simulink model "rpoco8_100_r2"  (R2013a)
settings: Solver=VariableStepDiscrete  SolverMode=SingleTasking  StartTime=0.0  StopTime=10.0  RelTol=1e-3
libraries: xbsIndex_r4 x2263, casper_library_misc x52, casper_library_multipliers x19, xps_library x5, casper_library_sources x4, casper_library_delays x1
(part 3 of 27)

== system rpoco8_100_r2/eq_fft3 ==
  note: Slice out 6 MSb of addr counter
      | to select 32 coeffs per antenna's (2) N fft bins
  pol1 : Inport
  sync : Inport  Port=2
  coeff : Inport  Port=3
  coeff_we : Inport  Port=4
  coeff_addr : Inport  Port=5
  Constant4 : xbsIndex_r4/Constant  const=0  gui_display_data_type=Fixed-point  arith_type=Unsigned  n_bits=17  bin_pt=7  preci_type=Single  exp_width=8  frac_width=24  explicit_period=on  period=1  equ=P=C  opselect=C  inp2=PCIN>>17  opr=+  inp1=P  carry=CIN  dbl_ovrd=off  block_type=constant
  Constant5 : xbsIndex_r4/Constant  const=0  gui_display_data_type=Fixed-point  arith_type=Boolean  n_bits=1  bin_pt=0  preci_type=Single  exp_width=8  frac_width=24  explicit_period=on  period=1  equ=P=C  opselect=C  inp2=PCIN>>17  opr=+  inp1=P  carry=CIN  dbl_ovrd=off  block_type=constant
  Counter2 : xbsIndex_r4/Counter  cnt_type=Free Running  cnt_to=Inf  operation=Up  start_count=0  cnt_by_val=1  arith_type=Unsigned  n_bits=nchan  bin_pt=0  load_pin=off  rst=on  en=off  explicit_period=off  period=1  dbl_ovrd=off  use_behavioral_HDL=off  implementation=Fabric  use_rpm=on  block_type=counter
      settings: xl_area=[0, 0, 0, 0, 0, 0, 0]
  Delay11 : xbsIndex_r4/Delay  rst=off  infoeditControl=Selection of Reset will increase slice count due to use of real FFs and instead of SRLs  en=off  latency=2  dbl_ovrd=off  reg_retiming=off  block_type=delay
      settings: xl_area=[0, 0, 0, 0, 0, 0, 0]
  Delay4 : xbsIndex_r4/Delay  rst=off  infoeditControl=Selection of Reset will increase slice count due to use of real FFs and instead of SRLs  en=off  latency=7  dbl_ovrd=off  reg_retiming=off  block_type=delay
      settings: xl_area=[0, 0, 0, 0, 0, 0, 0]
  Dual Port RAM : xbsIndex_r4/Dual Port RAM  depth=2^6  initVector=0  distributed_mem=Block RAM  init_a=0  init_b=0  rst_a=off  rst_b=off  en_a=off  en_b=off  latency=2  write_mode_A=Read After Write  write_mode_B=Read After Write  dbl_ovrd=off  optimize=Area  block_type=dpram
      settings: xl_area=[0, 0, 0, 0, 0, 0, 0]  block_version=10.1.3
  Reinterpret1 : xbsIndex_r4/Reinterpret  force_arith_type=on  arith_type=Unsigned  force_bin_pt=on  bin_pt=7  block_type=reinterpret
      settings: infoedit="Changes signal type without altering the binary representation.   You can changed the signal between signed and unsigned, and relocate the binary point.<br><br>Hardware notes: In hardware this block costs nothing.<br><br>Example:  Suppose the input is 6 bits wide, signed, with 2 fractional bits, and the output is forced to unsigned with 0 fractional bits.  Then an input of -2.0 (1110.00 in binary 2's complement) becomes an output of 56 (111000 in binary)."  block_version=10.1.3
  Slice : xbsIndex_r4/Slice  nbits=6  boolean_output=off  mode=Upper Bit Location + Width  bit1=0  base1=MSB of Input  bit0=0  base0=LSB of Input  dbl_ovrd=off  block_type=slice
      settings: infoedit="Extracts a given range of bits from each input sample and presents it at the output.  The output type is ordinarily unsigned with binary point at zero, but can be Boolean when the slice is one bit wide.<P><P>Hardware notes: In hardware this block costs nothing."  block_version=10.1.3
  Terminator : Terminator
  round1 : Subsystem  mask{n_bits=18}
      mask prompts: n_bits "Output Bitwidth"
  dout : Outport
  sync_out : Outport  Port=2
  clip : Outport  Port=3
  wires:
  Constant4/1 -> Dual Port RAM/2
  Constant5/1 -> Dual Port RAM/3
  coeff_addr/1 -> Dual Port RAM/4
  coeff_we/1 -> Dual Port RAM/6
  Reinterpret1/1 -> Dual Port RAM/5
  sync/1 -> Counter2/1, Delay4/1
  coeff/1 -> Reinterpret1/1
  round1/1(dout) -> dout/1
  Delay11/1 -> round1/1(din)
  pol1/1 -> Delay11/1
  Delay4/1 -> sync_out/1
  round1/2(clip) -> clip/1
  Counter2/1 -> Slice/1
  Slice/1 -> Dual Port RAM/1
  Dual Port RAM/2 -> Terminator/1
  Dual Port RAM/1 -> round1/2(scale)

== system rpoco8_100_r2/fft_pol02_imag ==
  addr : Inport
  data_in : Inport  Port=2
  we : Inport  Port=3
  calc_add : Subsystem  mask{data_width=32, addr_width=11, sample_rate=sample_rate}
      mask prompts: data_width "data width"; addr_width "address width"; sample_rate "sample rate"
  convert_addr : xbsIndex_r4/Convert  gui_display_data_type=Fixed-point  arith_type=Unsigned  n_bits=addr_width  bin_pt=0  float_type=Single  exp_bits=8  fraction_bits=24  quantization=Truncate  overflow=Wrap  en=off  latency=0  dbl_ovrd=off  pipeline=off  block_type=convert
      settings: xl_area=[0, 0, 0, 0, 0, 0, 0]
  convert_din1 : xbsIndex_r4/Convert  gui_display_data_type=Fixed-point  arith_type=Unsigned  n_bits=32  bin_pt=0  float_type=Single  exp_bits=8  fraction_bits=24  quantization=Truncate  overflow=Wrap  en=off  latency=0  dbl_ovrd=off  pipeline=off  block_type=convert
      settings: xl_area=[0, 0, 0, 0, 0, 0, 0]
  convert_we : xbsIndex_r4/Convert  gui_display_data_type=Fixed-point  arith_type=Unsigned  n_bits=1  bin_pt=0  float_type=Single  exp_bits=8  fraction_bits=24  quantization=Truncate  overflow=Wrap  en=off  latency=0  dbl_ovrd=off  pipeline=off  block_type=convert
      settings: xl_area=[0, 0, 0, 0, 0, 0, 0]
  mem : Subsystem
  munge_in : Subsystem  AncestorBlock=casper_library_flow_control/munge  mask(munge){divisions=1, div_size=32, order=[0], arith_type_out=Unsigned, bin_pt_out=0}
      mask prompts: divisions "Number of divisions"; div_size "Division size (bits)"; order "Division packing order"; arith_type_out "Output arithmetic type"; bin_pt_out "Output binary point"
      mask help: Splits an input bus into the specified number of divisions and then recombines them in the order specified (most significant division = 0,least = number divisions-1)
      mask init:
      | munge_init(gcb, ...
      |     'divisions', divisions, ...
      |     'div_size', div_size, ...
      |     'order', order, ...
      |     'arith_type_out', arith_type_out, ...
      |     'bin_pt_out', bin_pt_out);
      settings: AttributesFormatString=|
      | split:32
      | join:0
      | Unsigned [32,0]
      mask TypeOptions arith_type_out: Unsigned | Signed  (2's comp) | Floating-point
  munge_out : Subsystem  AncestorBlock=casper_library_flow_control/munge  mask(munge){divisions=1, div_size=32, order=[0], arith_type_out=Unsigned, bin_pt_out=0}
      mask prompts: divisions "Number of divisions"; div_size "Division size (bits)"; order "Division packing order"; arith_type_out "Output arithmetic type"; bin_pt_out "Output binary point"
      mask help: Splits an input bus into the specified number of divisions and then recombines them in the order specified (most significant division = 0,least = number divisions-1)
      mask init:
      | munge_init(gcb, ...
      |     'divisions', divisions, ...
      |     'div_size', div_size, ...
      |     'order', order, ...
      |     'arith_type_out', arith_type_out, ...
      |     'bin_pt_out', bin_pt_out);
      settings: AttributesFormatString=|
      | split:32
      | join:0
      | Unsigned [32,0]
      mask TypeOptions arith_type_out: Unsigned | Signed  (2's comp) | Floating-point
  rpoco8_r2_fft_pol02_imag_addr : xbsIndex_r4/Gateway Out  inherit_from_input=off  hdl_port=on  timing_constraint=None  locs_specified=off  LOCs={'A5','B9','A9','C1','A3','G6','E9','A6','A7','A8','B8','B1','B3','D9','B5','B4','B6','C2'}  UseAsDAC=off  DACChannel='1'  block_type=gatewayout
      settings: infoedit="Gateway out block.  Converts Xilinx fixed point inputs into ouputs of type Simulink integer, double, or fixed point.<P><P>Hardware notes:  In hardware these blocks become top level output ports or are discarded, depending on how they are configured."  xl_area=[0, 0, 0, 0, 0, 0, 0]  sginterface={'Nallatech'=>{'xdspkit'=>{'non_memory_mapped_port'=>'uprev_Shared_BRAM_addr'}},'Xilinx'=>{'jtaghwcosim'=>{'non_memory_mapped_port'=>'uprev_Shared_BRAM_addr'},'xdspkit'=>{'non_memory_mapped_port'=>'uprev_Shared_BRAM_addr'}}}
  rpoco8_r2_fft_pol02_imag_data_in : xbsIndex_r4/Gateway Out  inherit_from_input=off  hdl_port=on  timing_constraint=None  locs_specified=off  LOCs={'B21','B22','A22','B23','B19','C19','A20','A21','A23','B24','A24','A25','E18','D18','C18','B18'}  UseAsDAC=off  DACChannel='1'  block_type=gatewayout
      settings: infoedit="Gateway out block.  Converts Xilinx fixed point inputs into ouputs of type Simulink integer, double, or fixed point.<P><P>Hardware notes:  In hardware these blocks become top level output ports or are discarded, depending on how they are configured."  xl_area=[0, 0, 0, 0, 0, 0, 0]  sginterface={'Nallatech'=>{'xdspkit'=>{'non_memory_mapped_port'=>'uprev_Shared_BRAM_data_in'}},'Xilinx'=>{'jtaghwcosim'=>{'non_memory_mapped_port'=>'uprev_Shared_BRAM_data_in'},'xdspkit'=>{'non_memory_mapped_port'=>'uprev_Shared_BRAM_data_in'}}}
  rpoco8_r2_fft_pol02_imag_data_out : xbsIndex_r4/Gateway In  gui_display_data_type=Fixed-point  arith_type=Unsigned  n_bits=32  bin_pt=0  preci_type=Single  exp_width=8  frac_width=24  quantization=Truncate  overflow=Wrap  period=sample_rate  dbl_ovrd=off  timing_constraint=None  locs_specified=off  LOCs={}  UseAsADC=off  ADCChannel='1'  inherit_from_input=off  hdl_port=on  block_type=gatewayin
      settings: xl_area=[0, 0, 0, 0, 0, 0, 0]
  rpoco8_r2_fft_pol02_imag_we : xbsIndex_r4/Gateway Out  inherit_from_input=off  hdl_port=on  timing_constraint=None  locs_specified=off  LOCs={'A14'}  UseAsDAC=off  DACChannel='1'  block_type=gatewayout
      settings: infoedit="Gateway out block.  Converts Xilinx fixed point inputs into ouputs of type Simulink integer, double, or fixed point.<P><P>Hardware notes:  In hardware these blocks become top level output ports or are discarded, depending on how they are configured."  xl_area=[0, 0, 0, 0, 0, 0, 0]
  data_out : Outport
  wires:
  convert_addr/1 -> rpoco8_r2_fft_pol02_imag_addr/1
  convert_din1/1 -> rpoco8_r2_fft_pol02_imag_data_in/1
  data_in/1 -> munge_in/1(din)
  calc_add/1(out) -> convert_addr/1
  rpoco8_r2_fft_pol02_imag_we/1 -> mem/3(In3)
  rpoco8_r2_fft_pol02_imag_data_in/1 -> mem/2(In2)
  rpoco8_r2_fft_pol02_imag_addr/1 -> mem/1(In1)
  convert_we/1 -> rpoco8_r2_fft_pol02_imag_we/1
  rpoco8_r2_fft_pol02_imag_data_out/1 -> munge_out/1(din)
  mem/1(Out1) -> rpoco8_r2_fft_pol02_imag_data_out/1
  addr/1 -> calc_add/1(in)
  we/1 -> convert_we/1
  munge_out/1(dout) -> data_out/1
  munge_in/1(dout) -> convert_din1/1

== system rpoco8_100_r2/fft_pol02_real ==
  addr : Inport
  data_in : Inport  Port=2
  we : Inport  Port=3
  calc_add : Subsystem  mask{data_width=32, addr_width=11, sample_rate=sample_rate}
      mask prompts: data_width "data width"; addr_width "address width"; sample_rate "sample rate"
  convert_addr : xbsIndex_r4/Convert  gui_display_data_type=Fixed-point  arith_type=Unsigned  n_bits=addr_width  bin_pt=0  float_type=Single  exp_bits=8  fraction_bits=24  quantization=Truncate  overflow=Wrap  en=off  latency=0  dbl_ovrd=off  pipeline=off  block_type=convert
      settings: xl_area=[0, 0, 0, 0, 0, 0, 0]
  convert_din1 : xbsIndex_r4/Convert  gui_display_data_type=Fixed-point  arith_type=Unsigned  n_bits=32  bin_pt=0  float_type=Single  exp_bits=8  fraction_bits=24  quantization=Truncate  overflow=Wrap  en=off  latency=0  dbl_ovrd=off  pipeline=off  block_type=convert
      settings: xl_area=[0, 0, 0, 0, 0, 0, 0]
  convert_we : xbsIndex_r4/Convert  gui_display_data_type=Fixed-point  arith_type=Unsigned  n_bits=1  bin_pt=0  float_type=Single  exp_bits=8  fraction_bits=24  quantization=Truncate  overflow=Wrap  en=off  latency=0  dbl_ovrd=off  pipeline=off  block_type=convert
      settings: xl_area=[0, 0, 0, 0, 0, 0, 0]
  mem : Subsystem
  munge_in : Subsystem  AncestorBlock=casper_library_flow_control/munge  mask(munge){divisions=1, div_size=32, order=[0], arith_type_out=Unsigned, bin_pt_out=0}
      mask prompts: divisions "Number of divisions"; div_size "Division size (bits)"; order "Division packing order"; arith_type_out "Output arithmetic type"; bin_pt_out "Output binary point"
      mask help: Splits an input bus into the specified number of divisions and then recombines them in the order specified (most significant division = 0,least = number divisions-1)
      mask init:
      | munge_init(gcb, ...
      |     'divisions', divisions, ...
      |     'div_size', div_size, ...
      |     'order', order, ...
      |     'arith_type_out', arith_type_out, ...
      |     'bin_pt_out', bin_pt_out);
      settings: AttributesFormatString=|
      | split:32
      | join:0
      | Unsigned [32,0]
      mask TypeOptions arith_type_out: Unsigned | Signed  (2's comp) | Floating-point
  munge_out : Subsystem  AncestorBlock=casper_library_flow_control/munge  mask(munge){divisions=1, div_size=32, order=[0], arith_type_out=Unsigned, bin_pt_out=0}
      mask prompts: divisions "Number of divisions"; div_size "Division size (bits)"; order "Division packing order"; arith_type_out "Output arithmetic type"; bin_pt_out "Output binary point"
      mask help: Splits an input bus into the specified number of divisions and then recombines them in the order specified (most significant division = 0,least = number divisions-1)
      mask init:
      | munge_init(gcb, ...
      |     'divisions', divisions, ...
      |     'div_size', div_size, ...
      |     'order', order, ...
      |     'arith_type_out', arith_type_out, ...
      |     'bin_pt_out', bin_pt_out);
      settings: AttributesFormatString=|
      | split:32
      | join:0
      | Unsigned [32,0]
      mask TypeOptions arith_type_out: Unsigned | Signed  (2's comp) | Floating-point
  rpoco8_r2_fft_pol02_real_addr : xbsIndex_r4/Gateway Out  inherit_from_input=off  hdl_port=on  timing_constraint=None  locs_specified=off  LOCs={'A5','B9','A9','C1','A3','G6','E9','A6','A7','A8','B8','B1','B3','D9','B5','B4','B6','C2'}  UseAsDAC=off  DACChannel='1'  block_type=gatewayout
      settings: infoedit="Gateway out block.  Converts Xilinx fixed point inputs into ouputs of type Simulink integer, double, or fixed point.<P><P>Hardware notes:  In hardware these blocks become top level output ports or are discarded, depending on how they are configured."  xl_area=[0, 0, 0, 0, 0, 0, 0]  sginterface={'Nallatech'=>{'xdspkit'=>{'non_memory_mapped_port'=>'uprev_Shared_BRAM_addr'}},'Xilinx'=>{'jtaghwcosim'=>{'non_memory_mapped_port'=>'uprev_Shared_BRAM_addr'},'xdspkit'=>{'non_memory_mapped_port'=>'uprev_Shared_BRAM_addr'}}}
  rpoco8_r2_fft_pol02_real_data_in : xbsIndex_r4/Gateway Out  inherit_from_input=off  hdl_port=on  timing_constraint=None  locs_specified=off  LOCs={'B21','B22','A22','B23','B19','C19','A20','A21','A23','B24','A24','A25','E18','D18','C18','B18'}  UseAsDAC=off  DACChannel='1'  block_type=gatewayout
      settings: infoedit="Gateway out block.  Converts Xilinx fixed point inputs into ouputs of type Simulink integer, double, or fixed point.<P><P>Hardware notes:  In hardware these blocks become top level output ports or are discarded, depending on how they are configured."  xl_area=[0, 0, 0, 0, 0, 0, 0]  sginterface={'Nallatech'=>{'xdspkit'=>{'non_memory_mapped_port'=>'uprev_Shared_BRAM_data_in'}},'Xilinx'=>{'jtaghwcosim'=>{'non_memory_mapped_port'=>'uprev_Shared_BRAM_data_in'},'xdspkit'=>{'non_memory_mapped_port'=>'uprev_Shared_BRAM_data_in'}}}
  rpoco8_r2_fft_pol02_real_data_out : xbsIndex_r4/Gateway In  gui_display_data_type=Fixed-point  arith_type=Unsigned  n_bits=32  bin_pt=0  preci_type=Single  exp_width=8  frac_width=24  quantization=Truncate  overflow=Wrap  period=sample_rate  dbl_ovrd=off  timing_constraint=None  locs_specified=off  LOCs={}  UseAsADC=off  ADCChannel='1'  inherit_from_input=off  hdl_port=on  block_type=gatewayin
      settings: xl_area=[0, 0, 0, 0, 0, 0, 0]
  rpoco8_r2_fft_pol02_real_we : xbsIndex_r4/Gateway Out  inherit_from_input=off  hdl_port=on  timing_constraint=None  locs_specified=off  LOCs={'A14'}  UseAsDAC=off  DACChannel='1'  block_type=gatewayout
      settings: infoedit="Gateway out block.  Converts Xilinx fixed point inputs into ouputs of type Simulink integer, double, or fixed point.<P><P>Hardware notes:  In hardware these blocks become top level output ports or are discarded, depending on how they are configured."  xl_area=[0, 0, 0, 0, 0, 0, 0]
  data_out : Outport
  wires:
  convert_addr/1 -> rpoco8_r2_fft_pol02_real_addr/1
  convert_din1/1 -> rpoco8_r2_fft_pol02_real_data_in/1
  data_in/1 -> munge_in/1(din)
  calc_add/1(out) -> convert_addr/1
  rpoco8_r2_fft_pol02_real_we/1 -> mem/3(In3)
  rpoco8_r2_fft_pol02_real_data_in/1 -> mem/2(In2)
  rpoco8_r2_fft_pol02_real_addr/1 -> mem/1(In1)
  convert_we/1 -> rpoco8_r2_fft_pol02_real_we/1
  rpoco8_r2_fft_pol02_real_data_out/1 -> munge_out/1(din)
  mem/1(Out1) -> rpoco8_r2_fft_pol02_real_data_out/1
  addr/1 -> calc_add/1(in)
  we/1 -> convert_we/1
  munge_out/1(dout) -> data_out/1
  munge_in/1(dout) -> convert_din1/1

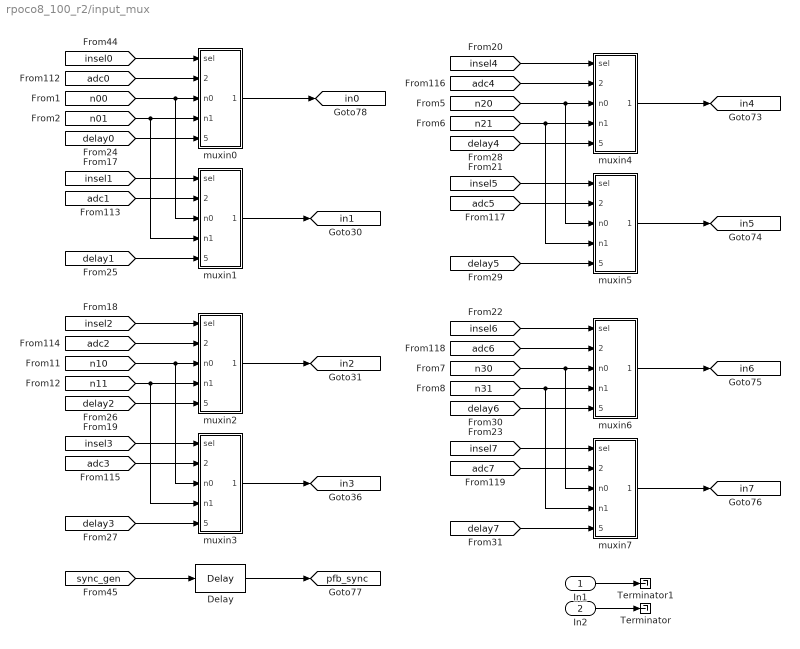
== system rpoco8_100_r2/input_mux ==
  In1 : Inport
  In2 : Inport  Port=2
  Delay : xbsIndex_r4/Delay  rst=off  infoeditControl=Selection of Reset will increase slice count due to use of real FFs and instead of SRLs  en=off  latency=2  dbl_ovrd=off  reg_retiming=off  block_type=delay
  Terminator : Terminator
  Terminator1 : Terminator
  muxin0 : Subsystem
  muxin1 : Subsystem
  muxin2 : Subsystem
  muxin3 : Subsystem
  muxin4 : Subsystem
  muxin5 : Subsystem
  muxin6 : Subsystem
  muxin7 : Subsystem
  tag scope: in0=global, in1=global, in2=global, in3=global, in4=global, in5=global, in6=global, in7=global, pfb_sync=global
  wires:
  [insel0] -> muxin0/1(sel)
  [adc0] -> muxin0/2(adc)
  [n00] -> muxin0/3(n0), muxin1/3(n0)
  [n01] -> muxin0/4(n1), muxin1/4(n1)
  [delay0] -> muxin0/5(delay)
  muxin0/1(out) -> [in0]
  [insel1] -> muxin1/1(sel)
  [adc1] -> muxin1/2(adc)
  [delay1] -> muxin1/5(delay)
  [insel2] -> muxin2/1(sel)
  [adc2] -> muxin2/2(adc)
  [n10] -> muxin3/3(n0), muxin2/3(n0)
  [n11] -> muxin3/4(n1), muxin2/4(n1)
  [delay2] -> muxin2/5(delay)
  [insel3] -> muxin3/1(sel)
  [adc3] -> muxin3/2(adc)
  [delay3] -> muxin3/5(delay)
  muxin1/1(out) -> [in1]
  muxin2/1(out) -> [in2]
  muxin3/1(out) -> [in3]
  [insel4] -> muxin4/1(sel)
  [adc4] -> muxin4/2(adc)
  [n20] -> muxin5/3(n0), muxin4/3(n0)
  [n21] -> muxin5/4(n1), muxin4/4(n1)
  [delay4] -> muxin4/5(delay)
  [insel5] -> muxin5/1(sel)
  [adc5] -> muxin5/2(adc)
  [delay5] -> muxin5/5(delay)
  [insel6] -> muxin6/1(sel)
  [adc6] -> muxin6/2(adc)
  [n30] -> muxin7/3(n0), muxin6/3(n0)
  [n31] -> muxin7/4(n1), muxin6/4(n1)
  [delay6] -> muxin6/5(delay)
  [insel7] -> muxin7/1(sel)
  [adc7] -> muxin7/2(adc)
  [delay7] -> muxin7/5(delay)
  muxin7/1(out) -> [in7]
  muxin4/1(out) -> [in4]
  muxin5/1(out) -> [in5]
  muxin6/1(out) -> [in6]
  [sync_gen] -> Delay/1
  Delay/1 -> [pfb_sync]
  In1/1 -> Terminator1/1
  In2/1 -> Terminator/1

== system rpoco8_100_r2/insel ==
  note: insel is a 32 bit input. every 4 bits represents a
      | selection input in the mux subsystem block. The inputs
      | are as follows:0=adc, 1=noise0, 2=noise1, 3=constant (0)
  BitBasher : xbsIndex_r4/BitBasher  bitexpr=|  display_expr=off  sr_1=1  arith_type1=Unsigned  bin_pt1=0  sr_2=2  arith_type2=Unsigned  bin_pt2=0  sr_3=3  arith_type3=Unsigned  bin_pt3=0  sr_4=4  arith_type4=Unsigned  bin_pt4=0  dbl_ovrd=off  block_type=bitbasher
      | <!DOCTYPE HTML PUBLIC "-//W3C//DTD HTML 4.0//EN" "http://www.w3.org/TR/REC-html40/strict.dtd">
      | <html><head><meta name="qrichtext" content="1" /><style type="text/css">
      | p, li { white-space: pre-wrap; }
      | </style></head><body style=" font-family:'Sans Serif'; font-size:9pt; font-weight:400; font-style:normal;">
      | <p style=" margin-top:12px; margin-bottom:12px; margin-left:0px; margin-right:0px; -qt-block-indent:0; text-indent:0px; font-family:'MS Shell Dlg'; font-size:8pt;">insel0={insel[1:0]}<br />insel1={insel[5:4]}<br />insel2={insel[9:8]}<br />insel3={insel[13:12]}</p></body></html>
      settings: block_version=10.1.3
  BitBasher1 : xbsIndex_r4/BitBasher  bitexpr=|  display_expr=off  sr_1=1  arith_type1=Unsigned  bin_pt1=0  sr_2=2  arith_type2=Unsigned  bin_pt2=0  sr_3=3  arith_type3=Unsigned  bin_pt3=0  sr_4=4  arith_type4=Unsigned  bin_pt4=0  dbl_ovrd=off  block_type=bitbasher
      | <html><head><meta name="qrichtext" content="1" /><style type="text/css">
      | p, li { white-space: pre-wrap; }
      | </style></head><body style=" font-family:'MS Shell Dlg 2'; font-size:8.25pt; font-weight:400; font-style:normal;">
      | <p style=" margin-top:12px; margin-bottom:12px; margin-left:0px; margin-right:0px; -qt-block-indent:0; text-indent:0px; font-family:'MS Shell Dlg'; font-size:8pt;">insel4={insel[17:16]}<br />insel5={insel[21:20]}<br />insel6={insel[25:24]}<br />insel7={insel[29:28]}</p></body></html>
      settings: block_version=10.1.3
  Constant : Constant  Value=858862385
  insel_data : Subsystem  Tag=xps:sw_reg  AncestorBlock=xps_library/software register  mask(swreg){mode=one value, io_dir=From Processor, io_delay=0, sample_period=1, names=reg, bitwidths=32, arith_types=0, bin_pts=0, sim_port=on, show_format=off}
      mask prompts: io_dir "I/O direction"; io_delay "I/O delay"; sample_period "Sample period"; names "Name:"; bitwidths "Bitwidth:"; arith_types "Type (ufix=0, fix=1, bool=2):"; bin_pts "Binary pt:"; sim_port "Provide sim input/output?"; show_format "Print format string?"
      mask init:
      | swreg_init(gcb)
      settings: AttributesFormatString=1input
      mask TypeOptions mode: one value | fields of equal size | fields of arbitrary size
      mask Callback mode: swreg_cb(gcb);
      mask TypeOptions io_dir: To Processor | From Processor
      mask Callback io_dir:
      | mask_enables = get_param(gcb, 'MaskEnables');
      | mask_names = get_param(gcb, 'MaskNames');
      | if strcmp(get_param(gcb, 'io_dir'), 'To Processor'),
      |     mask_enables{ismember(mask_names, 'sample_period')} = 'off';
      | else
      |     mask_enables{ismember(mask_names, 'sample_period')} = 'on';
      | end
      | set_param(gcb, 'MaskEnables', mask_enables);
      mask Callback bitwidths: swreg_maskcheck(gcb);
      mask Callback arith_types: [numios, ~, ~, ~, current_types] = swreg_maskcheck(gcb);
      mask Callback bin_pts: swreg_maskcheck(gcb);
  tag scope: insel0=global, insel1=global, insel2=global, insel3=global, insel4=global, insel5=global, insel6=global, insel7=global
  wires:
  BitBasher/1 -> [insel0]
  BitBasher/2 -> [insel1]
  BitBasher/3 -> [insel2]
  BitBasher/4 -> [insel3]
  BitBasher1/1 -> [insel4]
  BitBasher1/2 -> [insel5]
  BitBasher1/3 -> [insel6]
  BitBasher1/4 -> [insel7]
  insel_data/1(in_reg) -> BitBasher/1, BitBasher1/1
  Constant/1 -> insel_data/1(sim_1)

== system rpoco8_100_r2/mux_sel_pfb ==
  sim_1 : Inport
  io_delay : xbsIndex_r4/Delay  rst=off  infoeditControl=Selection of Reset will increase slice count due to use of real FFs and instead of SRLs  en=off  latency=0  dbl_ovrd=off  reg_retiming=on  block_type=delay
  reint1 : xbsIndex_r4/Reinterpret  force_arith_type=on  arith_type=Unsigned  force_bin_pt=on  bin_pt=0  block_type=reinterpret
  rpoco8_r2_mux_sel_pfb_user_data_out : xbsIndex_r4/Gateway In  gui_display_data_type=Fixed-point  arith_type=Unsigned  n_bits=32  bin_pt=0  preci_type=Single  exp_width=8  frac_width=24  quantization="Round  (unbiased: +/- Inf)"  overflow=Saturate  period=1  dbl_ovrd=off  timing_constraint=None  locs_specified=off  LOCs={}  UseAsADC=off  ADCChannel='1'  inherit_from_input=off  hdl_port=on  block_type=gatewayin
  slice_reg : xbsIndex_r4/Slice  nbits=32  boolean_output=off  mode=Lower Bit Location + Width  bit1=0  base1=MSB of Input  bit0=0  base0=LSB of Input  dbl_ovrd=off  block_type=slice
  in_reg : Outport
  wires:
  rpoco8_r2_mux_sel_pfb_user_data_out/1 -> io_delay/1
  sim_1/1 -> rpoco8_r2_mux_sel_pfb_user_data_out/1
  io_delay/1 -> slice_reg/1
  slice_reg/1 -> reint1/1
  reint1/1 -> in_reg/1

== system rpoco8_100_r2/mux_sel_pfb_sync ==
  sim_1 : Inport
  io_delay : xbsIndex_r4/Delay  rst=off  infoeditControl=Selection of Reset will increase slice count due to use of real FFs and instead of SRLs  en=off  latency=0  dbl_ovrd=off  reg_retiming=on  block_type=delay
  reint1 : xbsIndex_r4/Reinterpret  force_arith_type=on  arith_type=Unsigned  force_bin_pt=on  bin_pt=0  block_type=reinterpret
  rpoco8_r2_mux_sel_pfb_sync_user_data_out : xbsIndex_r4/Gateway In  gui_display_data_type=Fixed-point  arith_type=Unsigned  n_bits=32  bin_pt=0  preci_type=Single  exp_width=8  frac_width=24  quantization="Round  (unbiased: +/- Inf)"  overflow=Saturate  period=1  dbl_ovrd=off  timing_constraint=None  locs_specified=off  LOCs={}  UseAsADC=off  ADCChannel='1'  inherit_from_input=off  hdl_port=on  block_type=gatewayin
  slice_reg : xbsIndex_r4/Slice  nbits=32  boolean_output=off  mode=Lower Bit Location + Width  bit1=0  base1=MSB of Input  bit0=0  base0=LSB of Input  dbl_ovrd=off  block_type=slice
  in_reg : Outport
  wires:
  rpoco8_r2_mux_sel_pfb_sync_user_data_out/1 -> io_delay/1
  sim_1/1 -> rpoco8_r2_mux_sel_pfb_sync_user_data_out/1
  io_delay/1 -> slice_reg/1
  slice_reg/1 -> reint1/1
  reint1/1 -> in_reg/1

== system rpoco8_100_r2/new_raw_capture ==
  sim_1 : Inport
  io_delay : xbsIndex_r4/Delay  rst=off  infoeditControl=Selection of Reset will increase slice count due to use of real FFs and instead of SRLs  en=off  latency=0  dbl_ovrd=off  reg_retiming=on  block_type=delay
  reint1 : xbsIndex_r4/Reinterpret  force_arith_type=on  arith_type=Unsigned  force_bin_pt=on  bin_pt=0  block_type=reinterpret
  rpoco8_r2_new_raw_capture_user_data_out : xbsIndex_r4/Gateway In  gui_display_data_type=Fixed-point  arith_type=Unsigned  n_bits=32  bin_pt=0  preci_type=Single  exp_width=8  frac_width=24  quantization="Round  (unbiased: +/- Inf)"  overflow=Saturate  period=1  dbl_ovrd=off  timing_constraint=None  locs_specified=off  LOCs={}  UseAsADC=off  ADCChannel='1'  inherit_from_input=off  hdl_port=on  block_type=gatewayin
  slice_reg : xbsIndex_r4/Slice  nbits=32  boolean_output=off  mode=Lower Bit Location + Width  bit1=0  base1=MSB of Input  bit0=0  base0=LSB of Input  dbl_ovrd=off  block_type=slice
  in_reg : Outport
  wires:
  rpoco8_r2_new_raw_capture_user_data_out/1 -> io_delay/1
  sim_1/1 -> rpoco8_r2_new_raw_capture_user_data_out/1
  io_delay/1 -> slice_reg/1
  slice_reg/1 -> reint1/1
  reint1/1 -> in_reg/1

== system rpoco8_100_r2/new_raw_capture_trig ==
  sim_1 : Inport
  io_delay : xbsIndex_r4/Delay  rst=off  infoeditControl=Selection of Reset will increase slice count due to use of real FFs and instead of SRLs  en=off  latency=0  dbl_ovrd=off  reg_retiming=on  block_type=delay
  reint1 : xbsIndex_r4/Reinterpret  force_arith_type=on  arith_type=Unsigned  force_bin_pt=on  bin_pt=0  block_type=reinterpret
  rpoco8_r2_new_raw_capture_trig_user_data_out : xbsIndex_r4/Gateway In  gui_display_data_type=Fixed-point  arith_type=Unsigned  n_bits=32  bin_pt=0  preci_type=Single  exp_width=8  frac_width=24  quantization="Round  (unbiased: +/- Inf)"  overflow=Saturate  period=1  dbl_ovrd=off  timing_constraint=None  locs_specified=off  LOCs={}  UseAsADC=off  ADCChannel='1'  inherit_from_input=off  hdl_port=on  block_type=gatewayin
  slice_reg : xbsIndex_r4/Slice  nbits=32  boolean_output=off  mode=Lower Bit Location + Width  bit1=0  base1=MSB of Input  bit0=0  base0=LSB of Input  dbl_ovrd=off  block_type=slice
  in_reg : Outport
  wires:
  rpoco8_r2_new_raw_capture_trig_user_data_out/1 -> io_delay/1
  sim_1/1 -> rpoco8_r2_new_raw_capture_trig_user_data_out/1
  io_delay/1 -> slice_reg/1
  slice_reg/1 -> reint1/1
  reint1/1 -> in_reg/1

== system rpoco8_100_r2/ping ==
  out_reg : Inport
  assert_reg : xbsIndex_r4/Assert  assert_type=on  type_source=Explicitly  gui_display_data_type=Fixed-point  arith_type=Unsigned  n_bits=32  bin_pt=0  preci_type=Single  exp_width=8  frac_width=24  assert_rate=off  rate_source=Explicitly  period=1  output_port=on  block_type=assert
  cast_gw : xbsIndex_r4/Convert  gui_display_data_type=Fixed-point  arith_type=Unsigned  n_bits=32  bin_pt=0  float_type=Single  exp_bits=8  fraction_bits=24  quantization=Truncate  overflow=Wrap  en=off  latency=0  dbl_ovrd=off  pipeline=off  block_type=convert
  io_delay : xbsIndex_r4/Delay  rst=off  infoeditControl=Selection of Reset will increase slice count due to use of real FFs and instead of SRLs  en=off  latency=0  dbl_ovrd=off  reg_retiming=on  block_type=delay
  reint1 : xbsIndex_r4/Reinterpret  force_arith_type=on  arith_type=Unsigned  force_bin_pt=on  bin_pt=0  block_type=reinterpret
  rpoco8_r2_ping_user_data_in : xbsIndex_r4/Gateway Out  inherit_from_input=off  hdl_port=on  timing_constraint=None  locs_specified=off  LOCs={}  UseAsDAC=off  DACChannel='1'  block_type=gatewayout
  sim_out : Terminator
  wires:
  io_delay/1 -> cast_gw/1
  cast_gw/1 -> rpoco8_r2_ping_user_data_in/1
  rpoco8_r2_ping_user_data_in/1 -> sim_out/1
  out_reg/1 -> assert_reg/1
  assert_reg/1 -> reint1/1
  reint1/1 -> io_delay/1

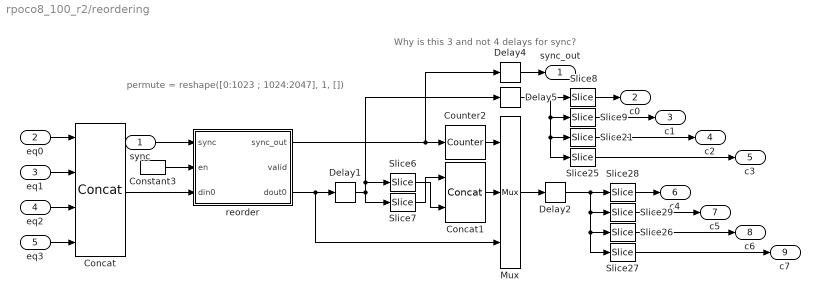
== system rpoco8_100_r2/reordering ==
  note: permute = reshape([0:1023 ; 1024:2047], 1, [])
  note: Why is this 3 and not 4 delays for sync?
  sync : Inport
  eq0 : Inport  Port=2
  eq1 : Inport  Port=3
  eq2 : Inport  Port=4
  eq3 : Inport  Port=5
  Concat : xbsIndex_r4/Concat  num_inputs=4  dbl_ovrd=off  block_type=concat
      settings: block_version=10.1.3
  Concat1 : xbsIndex_r4/Concat  num_inputs=2  dbl_ovrd=off  block_type=concat
      settings: block_version=10.1.3
  Constant3 : xbsIndex_r4/Constant  const=1  gui_display_data_type=Fixed-point  arith_type=Boolean  n_bits=16  bin_pt=14  preci_type=Single  exp_width=8  frac_width=24  explicit_period=on  period=1  equ=P=C  opselect=C  inp2=PCIN>>17  opr=+  inp1=P  carry=CIN  dbl_ovrd=off  block_type=constant
  Counter2 : xbsIndex_r4/Counter  cnt_type=Free Running  cnt_to=Inf  operation=Up  start_count=0  cnt_by_val=1  arith_type=Unsigned  n_bits=1  bin_pt=0  load_pin=off  rst=on  en=off  explicit_period=on  period=1  dbl_ovrd=off  use_behavioral_HDL=off  implementation=Fabric  use_rpm=on  block_type=counter
      settings: xl_area=[0, 0, 0, 0, 0, 0, 0]
  Delay1 : xbsIndex_r4/Delay  rst=off  infoeditControl=Selection of Reset will increase slice count due to use of real FFs and instead of SRLs  en=off  latency=2  dbl_ovrd=off  reg_retiming=on  block_type=delay
      settings: xl_area=[0, 0, 0, 0, 0, 0, 0]
  Delay2 : xbsIndex_r4/Delay  rst=off  infoeditControl=Selection of Reset will increase slice count due to use of real FFs and instead of SRLs  en=off  latency=1  dbl_ovrd=off  reg_retiming=on  block_type=delay
      settings: xl_area=[0, 0, 0, 0, 0, 0, 0]
  Delay4 : xbsIndex_r4/Delay  rst=off  infoeditControl=Selection of Reset will increase slice count due to use of real FFs and instead of SRLs  en=off  latency=4  dbl_ovrd=off  reg_retiming=on  block_type=delay
      settings: xl_area=[0, 0, 0, 0, 0, 0, 0]
  Delay5 : xbsIndex_r4/Delay  rst=off  infoeditControl=Selection of Reset will increase slice count due to use of real FFs and instead of SRLs  en=off  latency=2  dbl_ovrd=off  reg_retiming=on  block_type=delay
      settings: xl_area=[0, 0, 0, 0, 0, 0, 0]
  Mux : xbsIndex_r4/Mux  inputs=2  en=off  latency=2  precision=Full  arith_type=Unsigned  n_bits=16  bin_pt=14  quantization=Truncate  overflow=Wrap  dbl_ovrd=off  block_type=mux
  Slice21 : xbsIndex_r4/Slice  nbits=2*n_bits  boolean_output=off  mode=Upper Bit Location + Width  bit1=-4*n_bits  base1=MSB of Input  bit0=16  base0=LSB of Input  dbl_ovrd=off  block_type=slice
      settings: block_version=10.1.3
  Slice25 : xbsIndex_r4/Slice  nbits=2*n_bits  boolean_output=off  mode=Upper Bit Location + Width  bit1=-6*n_bits  base1=MSB of Input  bit0=16  base0=LSB of Input  dbl_ovrd=off  block_type=slice
      settings: block_version=10.1.3
  Slice26 : xbsIndex_r4/Slice  nbits=2*n_bits  boolean_output=off  mode=Upper Bit Location + Width  bit1=-4*n_bits  base1=MSB of Input  bit0=16  base0=LSB of Input  dbl_ovrd=off  block_type=slice
      settings: block_version=10.1.3
  Slice27 : xbsIndex_r4/Slice  nbits=2*n_bits  boolean_output=off  mode=Upper Bit Location + Width  bit1=-6*n_bits  base1=MSB of Input  bit0=16  base0=LSB of Input  dbl_ovrd=off  block_type=slice
      settings: block_version=10.1.3
  Slice28 : xbsIndex_r4/Slice  nbits=2*n_bits  boolean_output=off  mode=Upper Bit Location + Width  bit1=0  base1=MSB of Input  bit0=16  base0=LSB of Input  dbl_ovrd=off  block_type=slice
      settings: block_version=10.1.3
  Slice29 : xbsIndex_r4/Slice  nbits=2*n_bits  boolean_output=off  mode=Upper Bit Location + Width  bit1=-2*n_bits  base1=MSB of Input  bit0=16  base0=LSB of Input  dbl_ovrd=off  block_type=slice
      settings: block_version=10.1.3
  Slice6 : xbsIndex_r4/Slice  nbits=4*n_bits  boolean_output=off  mode=Upper Bit Location + Width  bit1=0  base1=MSB of Input  bit0=16  base0=LSB of Input  dbl_ovrd=off  block_type=slice
      settings: block_version=10.1.3
  Slice7 : xbsIndex_r4/Slice  nbits=4*n_bits  boolean_output=off  mode=Upper Bit Location + Width  bit1=-4*n_bits  base1=MSB of Input  bit0=16  base0=LSB of Input  dbl_ovrd=off  block_type=slice
      settings: block_version=10.1.3
  Slice8 : xbsIndex_r4/Slice  nbits=2*n_bits  boolean_output=off  mode=Upper Bit Location + Width  bit1=0  base1=MSB of Input  bit0=16  base0=LSB of Input  dbl_ovrd=off  block_type=slice
      settings: block_version=10.1.3
  Slice9 : xbsIndex_r4/Slice  nbits=2*n_bits  boolean_output=off  mode=Upper Bit Location + Width  bit1=-2*n_bits  base1=MSB of Input  bit0=16  base0=LSB of Input  dbl_ovrd=off  block_type=slice
      settings: block_version=10.1.3
  reorder : Subsystem  AncestorBlock=casper_library_reorder/reorder  mask(reorder){map=getfield( getfield( get_param( gcb,'UserData' ), 'parameters'),'map'), n_bits=0, n_inputs=1, bram_latency=2, map_latency=0, fanout_latency=0, double_buffer=0, bram_map=off}
      mask prompts: map "Output Order:"; n_bits "Data width in"; n_inputs "Number of inputs"; bram_latency "BRAM Latency"; map_latency "Map Latency"; fanout_latency "Fanout latency"; double_buffer "Double Buffer"; bram_map "Use BlockRAM for Map"
      mask init:
      | reorder_init(gcb, ...
      |     'map', map, ...
      |     'n_bits', n_bits, ...
      |     'n_inputs', n_inputs, ...
      |     'bram_latency', bram_latency, ...
      |     'map_latency', map_latency, ...
      |     'fanout_latency', fanout_latency, ...
      |     'double_buffer', double_buffer, ...
      |     'bram_map', bram_map);
      settings: AttributesFormatString=order=11
      mask Help: eval('xlWeb(''http://casper.berkeley.edu/wiki/Reorder'')')
  sync_out : Outport
  c0 : Outport  Port=2
  c1 : Outport  Port=3
  c2 : Outport  Port=4
  c3 : Outport  Port=5
  c4 : Outport  Port=6
  c5 : Outport  Port=7
  c6 : Outport  Port=8
  c7 : Outport  Port=9
  wires:
  Concat/1 -> reorder/3(din0)
  Constant3/1 -> reorder/2(en)
  Counter2/1 -> Mux/1
  reorder/1(sync_out) -> Counter2/1, Delay4/1
  reorder/3(dout0) -> Mux/3, Delay1/1
  Concat1/1 -> Mux/2
  Slice6/1 -> Concat1/2
  Slice7/1 -> Concat1/1
  Delay1/1 -> Slice7/1, Slice6/1, Delay5/1
  Mux/1 -> Delay2/1
  Delay5/1 -> Slice25/1, Slice21/1, Slice9/1, Slice8/1
  Delay4/1 -> sync_out/1
  Slice8/1 -> c0/1
  Slice9/1 -> c1/1
  eq0/1 -> Concat/1
  Slice21/1 -> c2/1
  sync/1 -> reorder/1(sync)
  Slice25/1 -> c3/1
  eq1/1 -> Concat/2
  Slice28/1 -> c4/1
  eq2/1 -> Concat/3
  Slice29/1 -> c5/1
  Slice26/1 -> c6/1
  eq3/1 -> Concat/4
  Slice27/1 -> c7/1
  Delay2/1 -> Slice28/1, Slice27/1, Slice26/1, Slice29/1

== system rpoco8_100_r2/seed ==
  BitBasher : xbsIndex_r4/BitBasher  bitexpr=|  display_expr=off  sr_1=1  arith_type1=Unsigned  bin_pt1=0  sr_2=2  arith_type2=Unsigned  bin_pt2=0  sr_3=3  arith_type3=Unsigned  bin_pt3=0  sr_4=4  arith_type4=Unsigned  bin_pt4=0  dbl_ovrd=off  block_type=bitbasher
      | <html><head><meta name="qrichtext" content="1" /><style type="text/css">
      | p, li { white-space: pre-wrap; }
      | </style></head><body style=" font-family:'MS Shell Dlg 2'; font-size:8.25pt; font-weight:400; font-style:normal;">
      | <p style=" margin-top:12px; margin-bottom:12px; margin-left:0px; margin-right:0px; -qt-block-indent:0; text-indent:0px; font-family:'MS Shell Dlg'; font-size:8pt;">seed0={8'h5c, seed[7:0], seed[0:7], 8'ha3}<br />seed1={8'h5c, seed[15:8], seed[8:15], 8'ha3}<br />seed2={8'h5c, seed[23:16], seed[16:23], 8'ha3}<br />seed3={8'h5c, seed[31:24], seed[24:31], 8'ha3}</p></body></html>
      settings: block_version=10.1.3
  Constant : Constant  Value=0
  armed_trigger : casper_library_misc/armed_trigger
  seed_data : Subsystem  Tag=xps:sw_reg  AncestorBlock=xps_library/software register  mask(swreg){mode=one value, io_dir=From Processor, io_delay=0, sample_period=1, names=reg, bitwidths=32, arith_types=0, bin_pts=0, sim_port=on, show_format=off}
      mask prompts: io_dir "I/O direction"; io_delay "I/O delay"; sample_period "Sample period"; names "Name:"; bitwidths "Bitwidth:"; arith_types "Type (ufix=0, fix=1, bool=2):"; bin_pts "Binary pt:"; sim_port "Provide sim input/output?"; show_format "Print format string?"
      mask init:
      | swreg_init(gcb)
      settings: AttributesFormatString=1input
      mask TypeOptions mode: one value | fields of equal size | fields of arbitrary size
      mask Callback mode: swreg_cb(gcb);
      mask TypeOptions io_dir: To Processor | From Processor
      mask Callback io_dir:
      | mask_enables = get_param(gcb, 'MaskEnables');
      | mask_names = get_param(gcb, 'MaskNames');
      | if strcmp(get_param(gcb, 'io_dir'), 'To Processor'),
      |     mask_enables{ismember(mask_names, 'sample_period')} = 'off';
      | else
      |     mask_enables{ismember(mask_names, 'sample_period')} = 'on';
      | end
      | set_param(gcb, 'MaskEnables', mask_enables);
      mask Callback bitwidths: swreg_maskcheck(gcb);
      mask Callback arith_types: [numios, ~, ~, ~, current_types] = swreg_maskcheck(gcb);
      mask Callback bin_pts: swreg_maskcheck(gcb);
  tag scope: seed0=global, seed1=global, seed2=global, seed3=global, seed_ld=global
  wires:
  BitBasher/1 -> [seed0]
  BitBasher/2 -> [seed1]
  BitBasher/3 -> [seed2]
  BitBasher/4 -> [seed3]
  seed_data/1(in_reg) -> BitBasher/1
  armed_trigger/1 -> [seed_ld]
  [sync_gen] -> armed_trigger/2
  Constant/1 -> seed_data/1(sim_1)
  [arm_rst] -> armed_trigger/1

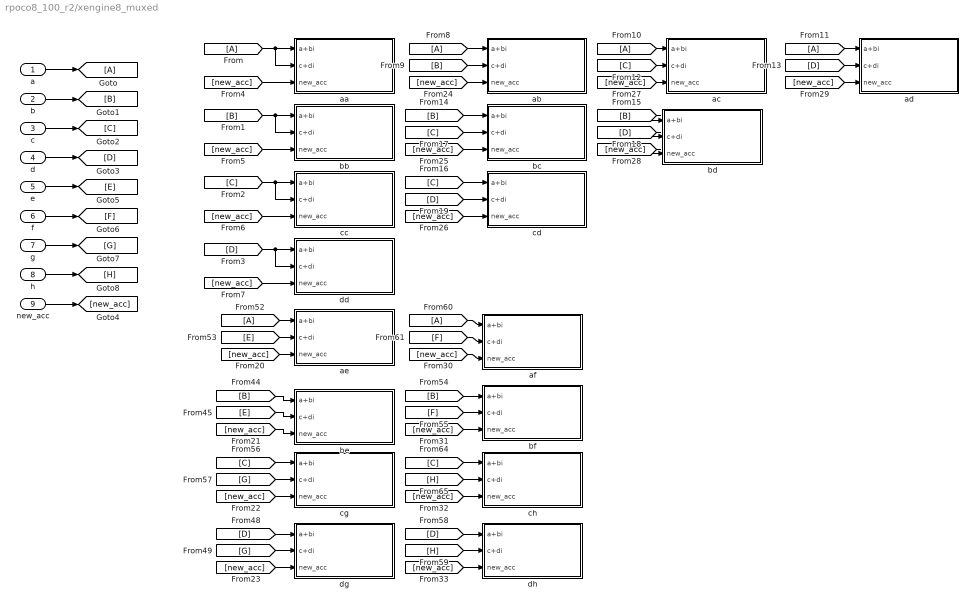
== system rpoco8_100_r2/xengine8_muxed ==
  a : Inport
  b : Inport  Port=2
  c : Inport  Port=3
  d : Inport  Port=4
  e : Inport  Port=5
  f : Inport  Port=6
  g : Inport  Port=7
  h : Inport  Port=8
  new_acc : Inport  Port=9
  aa : Subsystem
  ab : Subsystem
  ac : Subsystem
  ad : Subsystem
  ae : Subsystem
  af : Subsystem
  bb : Subsystem
  bc : Subsystem
  bd : Subsystem
  be : Subsystem
  bf : Subsystem
  cc : Subsystem
  cd : Subsystem
  cg : Subsystem
  ch : Subsystem
  dd : Subsystem
  dg : Subsystem
  dh : Subsystem
  wires:
  a/1 -> [A]
  b/1 -> [B]
  c/1 -> [C]
  d/1 -> [D]
  new_acc/1 -> [new_acc]
  [A] -> aa/2(c+di), aa/1(a+bi)
  [B] -> bb/1(a+bi), bb/2(c+di)
  [C] -> cc/1(a+bi), cc/2(c+di)
  [D] -> dd/1(a+bi), dd/2(c+di)
  [new_acc] -> aa/3(new_acc)
  [new_acc] -> bb/3(new_acc)
  [new_acc] -> cc/3(new_acc)
  [new_acc] -> dd/3(new_acc)
  [A] -> ac/1(a+bi)
  [A] -> ad/1(a+bi)
  [C] -> ac/2(c+di)
  [D] -> ad/2(c+di)
  [B] -> bc/1(a+bi)
  [B] -> bd/1(a+bi)
  [C] -> cd/1(a+bi)
  [C] -> bc/2(c+di)
  [D] -> bd/2(c+di)
  [D] -> cd/2(c+di)
  e/1 -> [E]
  f/1 -> [F]
  g/1 -> [G]
  h/1 -> [H]
  [B] -> be/1(a+bi)
  [E] -> be/2(c+di)
  [D] -> dg/1(a+bi)
  [G] -> dg/2(c+di)
  [A] -> ae/1(a+bi)
  [E] -> ae/2(c+di)
  [B] -> bf/1(a+bi)
  [F] -> bf/2(c+di)
  [C] -> cg/1(a+bi)
  [G] -> cg/2(c+di)
  [D] -> dh/1(a+bi)
  [H] -> dh/2(c+di)
  [A] -> af/1(a+bi)
  [F] -> af/2(c+di)
  [C] -> ch/1(a+bi)
  [H] -> ch/2(c+di)
  [new_acc] -> dg/3(new_acc)
  [new_acc] -> cg/3(new_acc)
  [new_acc] -> be/3(new_acc)
  [new_acc] -> ae/3(new_acc)
  [new_acc] -> cd/3(new_acc)
  [new_acc] -> bc/3(new_acc)
  [new_acc] -> bd/3(new_acc)
  [new_acc] -> ac/3(new_acc)
  [new_acc] -> ad/3(new_acc)
  [new_acc] -> af/3(new_acc)
  [new_acc] -> bf/3(new_acc)
  [new_acc] -> ch/3(new_acc)
  [new_acc] -> dh/3(new_acc)
  [new_acc] -> ab/3(new_acc)
  [A] -> ab/1(a+bi)
  [B] -> ab/2(c+di)

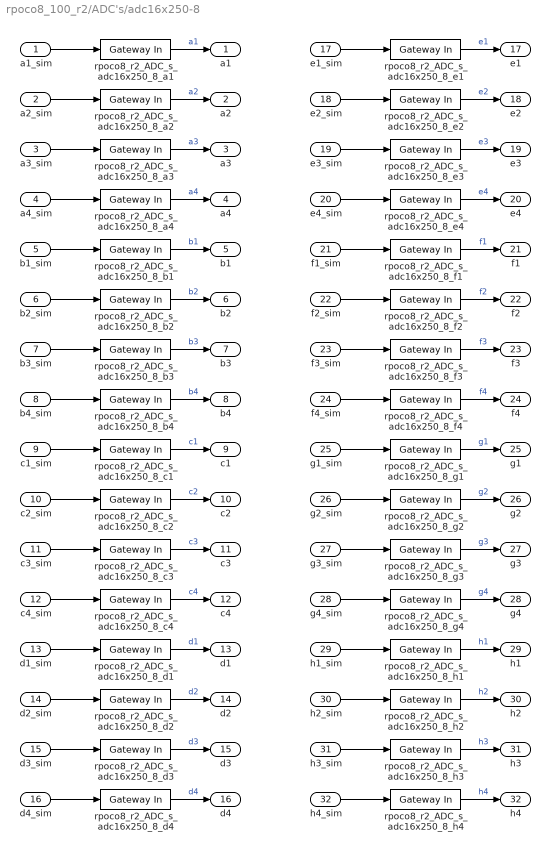
== system rpoco8_100_r2/ADC's/adc16x250-8 ==
  a1_sim : Inport
  a2_sim : Inport  Port=2
  a3_sim : Inport  Port=3
  a4_sim : Inport  Port=4
  b1_sim : Inport  Port=5
  b2_sim : Inport  Port=6
  b3_sim : Inport  Port=7
  b4_sim : Inport  Port=8
  c1_sim : Inport  Port=9
  c2_sim : Inport  Port=10
  c3_sim : Inport  Port=11
  c4_sim : Inport  Port=12
  d1_sim : Inport  Port=13
  d2_sim : Inport  Port=14
  d3_sim : Inport  Port=15
  d4_sim : Inport  Port=16
  e1_sim : Inport  Port=17
  e2_sim : Inport  Port=18
  e3_sim : Inport  Port=19
  e4_sim : Inport  Port=20
  f1_sim : Inport  Port=21
  f2_sim : Inport  Port=22
  f3_sim : Inport  Port=23
  f4_sim : Inport  Port=24
  g1_sim : Inport  Port=25
  g2_sim : Inport  Port=26
  g3_sim : Inport  Port=27
  g4_sim : Inport  Port=28
  h1_sim : Inport  Port=29
  h2_sim : Inport  Port=30
  h3_sim : Inport  Port=31
  h4_sim : Inport  Port=32
  rpoco8_r2_ADC_s_adc16x250_8_a{1..4} (4 alike) : xbsIndex_r4/Gateway In  gui_display_data_type=Fixed-point  arith_type="Signed  (2's comp)"  n_bits=8  bin_pt=7  preci_type=Single  exp_width=8  frac_width=24  quantization="Round  (unbiased: +/- Inf)"  overflow=Saturate  period=1  dbl_ovrd=off  timing_constraint=None  locs_specified=off  LOCs={}  UseAsADC=off  ADCChannel='1'  inherit_from_input=off  hdl_port=on  block_type=gatewayin
  rpoco8_r2_ADC_s_adc16x250_8_b{1..4} (4 alike) : xbsIndex_r4/Gateway In  gui_display_data_type=Fixed-point  arith_type="Signed  (2's comp)"  n_bits=8  bin_pt=7  preci_type=Single  exp_width=8  frac_width=24  quantization="Round  (unbiased: +/- Inf)"  overflow=Saturate  period=1  dbl_ovrd=off  timing_constraint=None  locs_specified=off  LOCs={}  UseAsADC=off  ADCChannel='1'  inherit_from_input=off  hdl_port=on  block_type=gatewayin
  rpoco8_r2_ADC_s_adc16x250_8_c{1..4} (4 alike) : xbsIndex_r4/Gateway In  gui_display_data_type=Fixed-point  arith_type="Signed  (2's comp)"  n_bits=8  bin_pt=7  preci_type=Single  exp_width=8  frac_width=24  quantization="Round  (unbiased: +/- Inf)"  overflow=Saturate  period=1  dbl_ovrd=off  timing_constraint=None  locs_specified=off  LOCs={}  UseAsADC=off  ADCChannel='1'  inherit_from_input=off  hdl_port=on  block_type=gatewayin
  rpoco8_r2_ADC_s_adc16x250_8_d{1..4} (4 alike) : xbsIndex_r4/Gateway In  gui_display_data_type=Fixed-point  arith_type="Signed  (2's comp)"  n_bits=8  bin_pt=7  preci_type=Single  exp_width=8  frac_width=24  quantization="Round  (unbiased: +/- Inf)"  overflow=Saturate  period=1  dbl_ovrd=off  timing_constraint=None  locs_specified=off  LOCs={}  UseAsADC=off  ADCChannel='1'  inherit_from_input=off  hdl_port=on  block_type=gatewayin
  rpoco8_r2_ADC_s_adc16x250_8_e{1..4} (4 alike) : xbsIndex_r4/Gateway In  gui_display_data_type=Fixed-point  arith_type="Signed  (2's comp)"  n_bits=8  bin_pt=7  preci_type=Single  exp_width=8  frac_width=24  quantization="Round  (unbiased: +/- Inf)"  overflow=Saturate  period=1  dbl_ovrd=off  timing_constraint=None  locs_specified=off  LOCs={}  UseAsADC=off  ADCChannel='1'  inherit_from_input=off  hdl_port=on  block_type=gatewayin
  rpoco8_r2_ADC_s_adc16x250_8_f{1..4} (4 alike) : xbsIndex_r4/Gateway In  gui_display_data_type=Fixed-point  arith_type="Signed  (2's comp)"  n_bits=8  bin_pt=7  preci_type=Single  exp_width=8  frac_width=24  quantization="Round  (unbiased: +/- Inf)"  overflow=Saturate  period=1  dbl_ovrd=off  timing_constraint=None  locs_specified=off  LOCs={}  UseAsADC=off  ADCChannel='1'  inherit_from_input=off  hdl_port=on  block_type=gatewayin
  rpoco8_r2_ADC_s_adc16x250_8_g{1..4} (4 alike) : xbsIndex_r4/Gateway In  gui_display_data_type=Fixed-point  arith_type="Signed  (2's comp)"  n_bits=8  bin_pt=7  preci_type=Single  exp_width=8  frac_width=24  quantization="Round  (unbiased: +/- Inf)"  overflow=Saturate  period=1  dbl_ovrd=off  timing_constraint=None  locs_specified=off  LOCs={}  UseAsADC=off  ADCChannel='1'  inherit_from_input=off  hdl_port=on  block_type=gatewayin
  rpoco8_r2_ADC_s_adc16x250_8_h{1..4} (4 alike) : xbsIndex_r4/Gateway In  gui_display_data_type=Fixed-point  arith_type="Signed  (2's comp)"  n_bits=8  bin_pt=7  preci_type=Single  exp_width=8  frac_width=24  quantization="Round  (unbiased: +/- Inf)"  overflow=Saturate  period=1  dbl_ovrd=off  timing_constraint=None  locs_specified=off  LOCs={}  UseAsADC=off  ADCChannel='1'  inherit_from_input=off  hdl_port=on  block_type=gatewayin
  a1 : Outport
  a2 : Outport  Port=2
  a3 : Outport  Port=3
  a4 : Outport  Port=4
  b1 : Outport  Port=5
  b2 : Outport  Port=6
  b3 : Outport  Port=7
  b4 : Outport  Port=8
  c1 : Outport  Port=9
  c2 : Outport  Port=10
  c3 : Outport  Port=11
  c4 : Outport  Port=12
  d1 : Outport  Port=13
  d2 : Outport  Port=14
  d3 : Outport  Port=15
  d4 : Outport  Port=16
  e1 : Outport  Port=17
  e2 : Outport  Port=18
  e3 : Outport  Port=19
  e4 : Outport  Port=20
  f1 : Outport  Port=21
  f2 : Outport  Port=22
  f3 : Outport  Port=23
  f4 : Outport  Port=24
  g1 : Outport  Port=25
  g2 : Outport  Port=26
  g3 : Outport  Port=27
  g4 : Outport  Port=28
  h1 : Outport  Port=29
  h2 : Outport  Port=30
  h3 : Outport  Port=31
  h4 : Outport  Port=32
  wires:
  a1_sim/1 -> rpoco8_r2_ADC_s_adc16x250_8_a1/1
  rpoco8_r2_ADC_s_adc16x250_8_a1/1 -> a1/1  "a1"
  a2_sim/1 -> rpoco8_r2_ADC_s_adc16x250_8_a2/1
  rpoco8_r2_ADC_s_adc16x250_8_a2/1 -> a2/1  "a2"
  a3_sim/1 -> rpoco8_r2_ADC_s_adc16x250_8_a3/1
  rpoco8_r2_ADC_s_adc16x250_8_a3/1 -> a3/1  "a3"
  a4_sim/1 -> rpoco8_r2_ADC_s_adc16x250_8_a4/1
  rpoco8_r2_ADC_s_adc16x250_8_a4/1 -> a4/1  "a4"
  b1_sim/1 -> rpoco8_r2_ADC_s_adc16x250_8_b1/1
  rpoco8_r2_ADC_s_adc16x250_8_b1/1 -> b1/1  "b1"
  b2_sim/1 -> rpoco8_r2_ADC_s_adc16x250_8_b2/1
  rpoco8_r2_ADC_s_adc16x250_8_b2/1 -> b2/1  "b2"
  b3_sim/1 -> rpoco8_r2_ADC_s_adc16x250_8_b3/1
  rpoco8_r2_ADC_s_adc16x250_8_b3/1 -> b3/1  "b3"
  b4_sim/1 -> rpoco8_r2_ADC_s_adc16x250_8_b4/1
  rpoco8_r2_ADC_s_adc16x250_8_b4/1 -> b4/1  "b4"
  c1_sim/1 -> rpoco8_r2_ADC_s_adc16x250_8_c1/1
  rpoco8_r2_ADC_s_adc16x250_8_c1/1 -> c1/1  "c1"
  c2_sim/1 -> rpoco8_r2_ADC_s_adc16x250_8_c2/1
  rpoco8_r2_ADC_s_adc16x250_8_c2/1 -> c2/1  "c2"
  c3_sim/1 -> rpoco8_r2_ADC_s_adc16x250_8_c3/1
  rpoco8_r2_ADC_s_adc16x250_8_c3/1 -> c3/1  "c3"
  c4_sim/1 -> rpoco8_r2_ADC_s_adc16x250_8_c4/1
  rpoco8_r2_ADC_s_adc16x250_8_c4/1 -> c4/1  "c4"
  d1_sim/1 -> rpoco8_r2_ADC_s_adc16x250_8_d1/1
  rpoco8_r2_ADC_s_adc16x250_8_d1/1 -> d1/1  "d1"
  d2_sim/1 -> rpoco8_r2_ADC_s_adc16x250_8_d2/1
  rpoco8_r2_ADC_s_adc16x250_8_d2/1 -> d2/1  "d2"
  d3_sim/1 -> rpoco8_r2_ADC_s_adc16x250_8_d3/1
  rpoco8_r2_ADC_s_adc16x250_8_d3/1 -> d3/1  "d3"
  d4_sim/1 -> rpoco8_r2_ADC_s_adc16x250_8_d4/1
  rpoco8_r2_ADC_s_adc16x250_8_d4/1 -> d4/1  "d4"
  e1_sim/1 -> rpoco8_r2_ADC_s_adc16x250_8_e1/1
  rpoco8_r2_ADC_s_adc16x250_8_e1/1 -> e1/1  "e1"
  e2_sim/1 -> rpoco8_r2_ADC_s_adc16x250_8_e2/1
  rpoco8_r2_ADC_s_adc16x250_8_e2/1 -> e2/1  "e2"
  e3_sim/1 -> rpoco8_r2_ADC_s_adc16x250_8_e3/1
  rpoco8_r2_ADC_s_adc16x250_8_e3/1 -> e3/1  "e3"
  e4_sim/1 -> rpoco8_r2_ADC_s_adc16x250_8_e4/1
  rpoco8_r2_ADC_s_adc16x250_8_e4/1 -> e4/1  "e4"
  f1_sim/1 -> rpoco8_r2_ADC_s_adc16x250_8_f1/1
  rpoco8_r2_ADC_s_adc16x250_8_f1/1 -> f1/1  "f1"
  f2_sim/1 -> rpoco8_r2_ADC_s_adc16x250_8_f2/1
  rpoco8_r2_ADC_s_adc16x250_8_f2/1 -> f2/1  "f2"
  f3_sim/1 -> rpoco8_r2_ADC_s_adc16x250_8_f3/1
  rpoco8_r2_ADC_s_adc16x250_8_f3/1 -> f3/1  "f3"
  f4_sim/1 -> rpoco8_r2_ADC_s_adc16x250_8_f4/1
  rpoco8_r2_ADC_s_adc16x250_8_f4/1 -> f4/1  "f4"
  g1_sim/1 -> rpoco8_r2_ADC_s_adc16x250_8_g1/1
  rpoco8_r2_ADC_s_adc16x250_8_g1/1 -> g1/1  "g1"
  g2_sim/1 -> rpoco8_r2_ADC_s_adc16x250_8_g2/1
  rpoco8_r2_ADC_s_adc16x250_8_g2/1 -> g2/1  "g2"
  g3_sim/1 -> rpoco8_r2_ADC_s_adc16x250_8_g3/1
  rpoco8_r2_ADC_s_adc16x250_8_g3/1 -> g3/1  "g3"
  g4_sim/1 -> rpoco8_r2_ADC_s_adc16x250_8_g4/1
  rpoco8_r2_ADC_s_adc16x250_8_g4/1 -> g4/1  "g4"
  h1_sim/1 -> rpoco8_r2_ADC_s_adc16x250_8_h1/1
  rpoco8_r2_ADC_s_adc16x250_8_h1/1 -> h1/1  "h1"
  h2_sim/1 -> rpoco8_r2_ADC_s_adc16x250_8_h2/1
  rpoco8_r2_ADC_s_adc16x250_8_h2/1 -> h2/1  "h2"
  h3_sim/1 -> rpoco8_r2_ADC_s_adc16x250_8_h3/1
  rpoco8_r2_ADC_s_adc16x250_8_h3/1 -> h3/1  "h3"
  h4_sim/1 -> rpoco8_r2_ADC_s_adc16x250_8_h4/1
  rpoco8_r2_ADC_s_adc16x250_8_h4/1 -> h4/1  "h4"
